simulink model "assembled"  (R2018b)
settings: Solver=FixedStepAuto  StartTime=0.0  StopTime=2500  FixedStep=sampletime  RelTol=1e-3
undefined symbols (not defined in the file or in its folder): Af, alfa, cd, fl, g, k, m, ro, sigbuilder_block
settings Model: Creator=Lac  LastModifiedBy=Lac

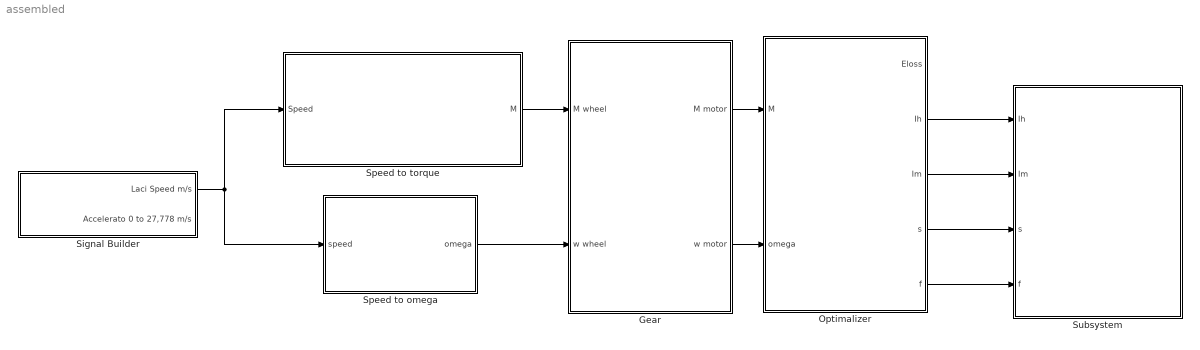
== system assembled ==
  Gear : Subsystem
  Optimalizer : Subsystem
  Signal Builder : Subsystem  Tag=STV Subsys  LoadFcn=sigbuilder_block('load');  StartFcn=sigbuilder_block('start');  StopFcn=sigbuilder_block('stop');  ClipboardFcn=sigbuilder_block('clipboard');  mask(Sigbuilder block){tuvar=[0:10]}
      mask help: Simulink:masks:SigbuilderBlock_MD
      mask init:
      | if ~strcmp(get_param(bdroot(gcbh),'SimulationStatus'),'stopped') tuvar = sigbuilder_block('maskInit'); end
      settings: CopyFcn=sigbuilder_block('copy');  DeleteFcn=sigbuilder_block('delete');  ModelCloseFcn=sigbuilder_block('modelClose');  PreSaveFcn=sigbuilder_block('preSave');  PauseFcn=sigbuilder_block('pause');  ContinueFcn=sigbuilder_block('continue');  NameChangeFcn=sigbuilder_block('namechange');  OpenFcn=sigbuilder_block('open',[5.4 30 1141.2 522.6 ]);  CloseFcn=sigbuilder_block('close');
      mask Display: plot(0, 0, 100, 100,[2, 2, 32, 32, 2], [68, 8, 8, 68, 68],[32, 2], [38, 38], [32, 19, 2],[53, 60, 44], [32, 17, 17, 2],[16, 16, 31, 31]);txt = getActiveGroup(gcbh);text(2, 100, txt,'verticalAlignment', 'top');
  Speed to omega : Subsystem
  Speed to torque : Subsystem
  Subsystem : Subsystem
  wires:
  Signal Builder/1(Laci Speed m/s) -> Speed to torque/1("Speed "), Speed to omega/1(speed)
  Speed to omega/1(omega) -> Gear/2(w wheel)
  Speed to torque/1("M ") -> Gear/1(M wheel)
  Gear/1(M motor) -> Optimalizer/1(M)
  Gear/2("w motor ") -> Optimalizer/2(omega)
  Optimalizer/4(s) -> Subsystem/3(s)
  Optimalizer/5(f) -> Subsystem/4(f)
  Optimalizer/3(Im) -> Subsystem/2(Im)
  Optimalizer/2(Ih) -> Subsystem/1(Ih)

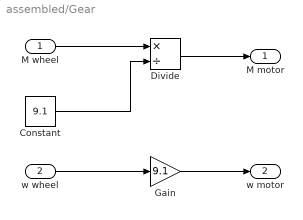
== system assembled/Gear ==
  M wheel : Inport
  w wheel : Inport  Port=2
  Constant : Constant  Value=9.1
  Divide : Product  Inputs=*/
  Gain : Gain  Gain=9.1
  M motor : Outport
  "w motor " : Outport  Port=2
  wires:
  Constant/1 -> Divide/2
  M wheel/1 -> Divide/1
  w wheel/1 -> Gain/1
  Gain/1 -> "w motor "/1
  Divide/1 -> M motor/1

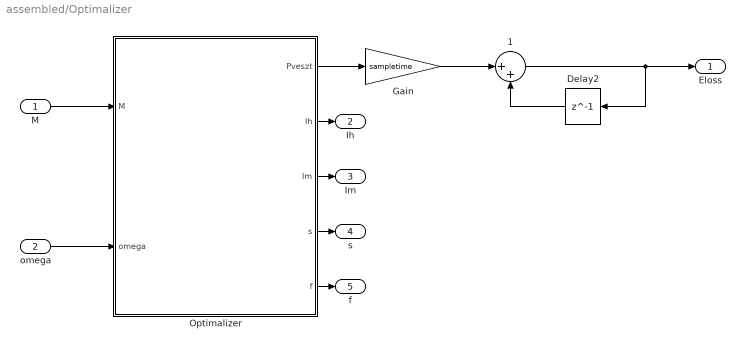
== system assembled/Optimalizer ==
  M : Inport
  omega : Inport  Port=2
  1 : Sum  Inputs=|++
  Delay2 : Delay  DelayLength=1  InitialCondition=0
  Gain : Gain  Gain=sampletime
  Optimalizer : MATLAB Function  TreatAsAtomicUnit=on
  Eloss : Outport
  Ih : Outport  Port=2
  Im : Outport  Port=3
  s : Outport  Port=4
  f : Outport  Port=5
  wires:
  Gain/1 -> 1/1
  Optimalizer/5(f) -> f/1
  Optimalizer/1(Pveszt) -> Gain/1
  Optimalizer/4(s) -> s/1
  omega/1 -> Optimalizer/2(omega)
  Optimalizer/3(Im) -> Im/1
  Optimalizer/2(Ih) -> Ih/1
  M/1 -> Optimalizer/1(M)
  1/1 -> Delay2/1, Eloss/1
  Delay2/1 -> 1/2

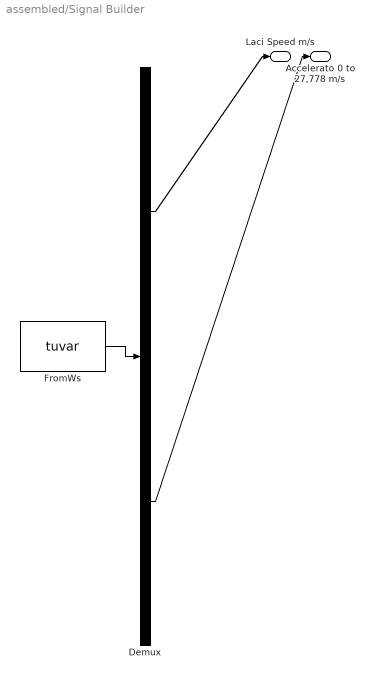
== system assembled/Signal Builder ==
  Demux : Demux  Tag=STV Demux  Outputs=2
  FromWs : FromWorkspace  Tag=STV FromWs  VariableName=tuvar  SampleTime=0
      SigBuilderData=|
      | common.afterFinalStr = 'Extrapolate'
      | common.sampleTime = 0
      | dataSet.timeRange = [0 7818]
      | dataSet.name = 'Group 1'
      | sbobj.Groups.Name = 'Group 1'
      | sbobj.Groups.Signals(1).Name = 'Laci Speed m/s'
      | sbobj.Groups.Signals(1).XData = [0 5 10 15 20 25 30 35 40 45 50 55 ... (483 elements, 1x483)]
      | sbobj.Groups.Signals(1).YData = [0 8.33333333333 8.33333333333 8.33333333333 8.33333333333 8.33333333333 8.33333333333 8.33333333333 8.33333333333 8.33333333333 8.33333333333 8.33333333333 ... (483 elements, 1x483)]
      | sbobj.Groups.Signals(2).Name = 'Accelerato 0 to 27,778 m/s'
      | sbobj.Groups.Signals(2).XData = [0 2.4 7818]
      | sbobj.Groups.Signals(2).YData = [0 27.7777777778 27.7777777778]
      | sbobj.Groups.TimeRange = [0 7818]
  Laci Speed m/s : Outport  Tag=STV Outport
  Accelerato 0 to 27,778 m/s : Outport  Tag=STV Outport  Port=2
  wires:
  FromWs/1 -> Demux/1
  Demux/1 -> Laci Speed m/s/1
  Demux/2 -> Accelerato 0 to 27,778 m/s/1

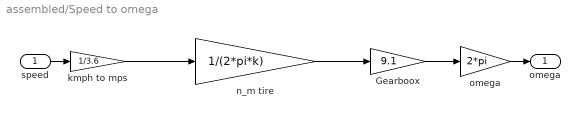
== system assembled/Speed to omega ==
  speed : Inport
  "Gearboox " : Gain  Gain=9.1
  kmph to mps : Gain  Gain=1/3.6
  "n_m tire " : Gain  Gain=1/(2*pi*k)
  "omega " : Gain  Gain=2*pi
  omega : Outport
  wires:
  speed/1 -> kmph to mps/1
  "n_m tire "/1 -> "Gearboox "/1
  "Gearboox "/1 -> "omega "/1
  kmph to mps/1 -> "n_m tire "/1
  "omega "/1 -> omega/1

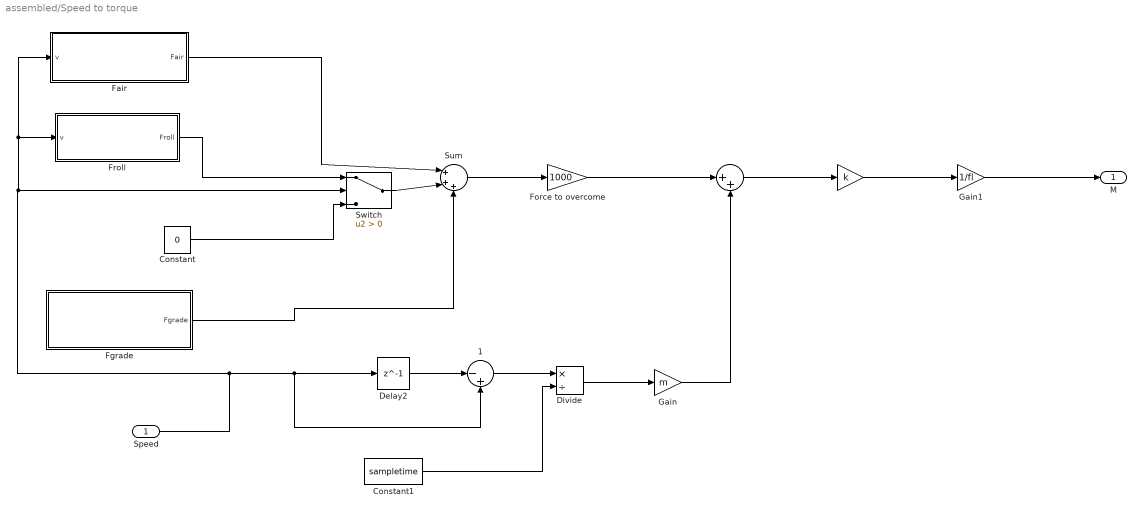
== system assembled/Speed to torque ==
  "Speed " : Inport
  " " : Gain  Gain=k
  " " : Sum  Inputs=|++
  " 1" : Sum  Inputs=|-+
  Constant : Constant  Value=0
  Constant1 : Constant  Value=sampletime
  Delay2 : Delay  DelayLength=1  InitialCondition=0
  Divide : Product  Inputs=*/
  "Fair " : Subsystem
  Fgrade : Subsystem
  Force to overcome : Gain  Gain=1000
  Froll : Subsystem
  Gain : Gain  Gain=m
  Gain1 : Gain  Gain=1/fl
  Sum : Sum  Inputs=|+++
  Switch : Switch  Criteria=u2 > Threshold
  "M " : Outport
  wires:
  "Fair "/1(Fair) -> Sum/1
  " 1"/1 -> Divide/1
  "Speed "/1 -> Delay2/1, " 1"/2, "Fair "/1(v), Froll/1(v), Switch/2
  Constant/1 -> Switch/3
  Sum/1 -> Force to overcome/1
  Switch/1 -> Sum/2
  Force to overcome/1 -> " "/1
  Delay2/1 -> " 1"/1
  Fgrade/1(Fgrade) -> Sum/3
  Divide/1 -> Gain/1
  Gain/1 -> " "/2
  Froll/1(Froll) -> Switch/1
  Constant1/1 -> Divide/2
  " "/1 -> " "/1
  Gain1/1 -> "M "/1
  " "/1 -> Gain1/1

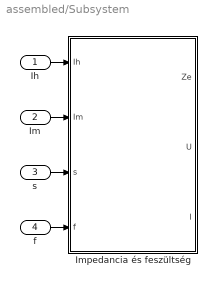
== system assembled/Subsystem ==
  Ih : Inport
  Im : Inport  Port=2
  s : Inport  Port=3
  f : Inport  Port=4
  "Impedancia és feszültség " : MATLAB Function  TreatAsAtomicUnit=on
  wires:
  s/1 -> "Impedancia és feszültség "/3(s)
  Im/1 -> "Impedancia és feszültség "/2(Im)
  f/1 -> "Impedancia és feszültség "/4(f)
  Ih/1 -> "Impedancia és feszültség "/1(Ih)

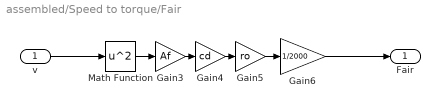
== system assembled/Speed to torque/Fair  ==
  v : Inport
  Gain3 : Gain  Gain=Af
  Gain4 : Gain  Gain=cd
  Gain5 : Gain  Gain=ro
  Gain6 : Gain  Gain=1/2000
  Math Function : Math  Operator=square  SaturateOnIntegerOverflow=on
  Fair : Outport
  wires:
  Math Function/1 -> Gain3/1
  Gain4/1 -> Gain5/1
  Gain3/1 -> Gain4/1
  Gain5/1 -> Gain6/1
  v/1 -> Math Function/1
  Gain6/1 -> Fair/1

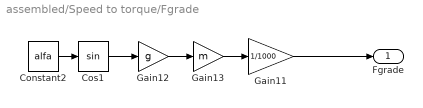
== system assembled/Speed to torque/Fgrade ==
  Constant2 : Constant  Value=alfa
  Cos1 : Trigonometry
  Gain11 : Gain  Gain=1/1000
  Gain12 : Gain  Gain=g
  Gain13 : Gain  Gain=m
  Fgrade : Outport
  wires:
  Gain13/1 -> Gain11/1
  Constant2/1 -> Cos1/1
  Cos1/1 -> Gain12/1
  Gain12/1 -> Gain13/1
  Gain11/1 -> Fgrade/1

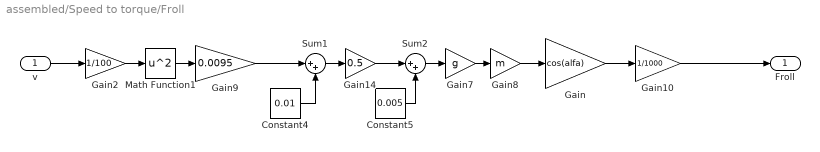
== system assembled/Speed to torque/Froll ==
  v : Inport
  Constant4 : Constant  Value=0.01
  Constant5 : Constant  Value=0.005
  Gain : Gain  Gain=cos(alfa)
  Gain10 : Gain  Gain=1/1000
  Gain14 : Gain  Gain=0.5
  Gain2 : Gain  Gain=1/100
  Gain7 : Gain  Gain=g
  Gain8 : Gain  Gain=m
  Gain9 : Gain  Gain=0.0095
  Math Function1 : Math  Operator=square  SaturateOnIntegerOverflow=on
  Sum1 : Sum  Inputs=|++
  Sum2 : Sum  Inputs=|++
  Froll : Outport
  wires:
  Gain8/1 -> Gain/1
  Constant4/1 -> Sum1/2
  Sum2/1 -> Gain7/1
  Gain9/1 -> Sum1/1
  Sum1/1 -> Gain14/1
  Gain10/1 -> Froll/1
  Constant5/1 -> Sum2/2
  Math Function1/1 -> Gain9/1
  Gain14/1 -> Sum2/1
  Gain7/1 -> Gain8/1
  Gain2/1 -> Math Function1/1
  v/1 -> Gain2/1
  Gain/1 -> Gain10/1

== matlab function assembled/Optimalizer/Optimalizer ==
  data: Pveszt output; Ih output; M input; omega input; Im output; s output; f output
function [Pveszt,Ih,Im,s,f]=optimal(M,omega)
p=1
Lm=0.0070547
R2=0.0072
%Pveszt szamolas, hogy egy megoldas legyen
a=Lm^4
b=-4*(Lm^3)*M*R2
c=((Lm^2)*4*(M^2)*(R2^2))-(8*(Lm^2)*(R2^2)*(M^2))
Pveszt1=((-b)+sqrt((b^2)-(4*a*c)))/(2*a)
Pveszt2=((-b)-sqrt((b^2)-(4*a*c)))/(2*a)
Pveszt=0;
if Pveszt1>0;
    Pveszt=Pveszt1;
elseif Pveszt2>0;
    Pveszt=Pveszt2;
end
a1=2*(Lm^2)*R2
b1=(Lm*2*M*R2)-(Pveszt*(Lm^2))
c1=(M^2)*R2
Ih=sqrt(abs(((-b1)+sqrt(complex((b1^2)-(4*a1*c1))))/(2*a1)))
Im=(M)/(Lm*Ih)
s=(((M*omega)/(3*R2*(Ih^2)))+1)^(-1)
n=(60*omega)/(2*pi)
f=-((n*p)/(60*(s-1)))

== matlab function assembled/Subsystem/Impedancia és feszültség  ==
  data: Ih input; Im input; s input; f input; Ze output; U output; I output
function [Ze,U,I]=ZU(Ih, Im, s, f)
Lm=0.0070547
Xm=Lm*2*pi*f
L2=0.0002406
R2=0.0072
X2=L2*2*pi*f
Rm=R2*((1-s)/s)
Z=(((1/(R2+(1i*X2)+Rm))+(1/(1i*Xm)))^(-1))+R2+(1i*X2)
Ze=abs(Z)
I=sqrt((Im^2)+(Ih^2))
U=I*Ze
